simulink model "detector13"  (Simulink 2.20)
settings: Solver=FixedStepDiscrete  StartTime=0.0  StopTime=30  RelTol=1e-3  AbsTol=1e-6
undefined symbols (not defined in the file): firls, get
libraries: BufferedDSP x22, dspbuff x7, dspsnks x2, dsparch x2, WinAudio x1
settings Model: SaveTime=off  SaveOutput=off  ConsistencyChecking=off  RTWPlaceOutputsASAP=off  RTWTemplateMakefile=c:\nfc\matlab\simulink\grt_vc_sgm.tmf  RTWMakeCommand="make_rtw USER_SRCS=\"winmm.lib\" USER_INCLUDES=\"-Ic:\\nfc\\matlab\\Simulink\\BufferedDSP\\src\\rtw\""

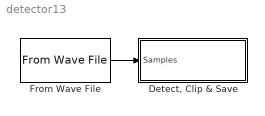
== system detector13 ==
  "Detect, Clip & Save" : Subsystem  mask(DetectClipNSave){buffersize=8192, f0=4100, f1=5500, threshold=2, numChannels=1, col_major=0, fs=22050}
      mask prompts: buffersize "Buffer Size:"; f0 "Lower Frequency (Hz):"; f1 "Upper Frequency (Hz):"; numChannels "Number of Channels:"; col_major "Column major channel order:"; fs "Sample Rate (Hz):"
      mask help: Detects acoustic events in a frequency band, clips, and saves them to disk.
      mask Help: Detects acoustic events in a frequency band, clips, and saves them to disk.
  From Wave File : WinAudio/From Wave File  sampleRate=22050  buffersize=8192  stereo=off  col_major=1  filename=c:\dicktest
  wires:
  From Wave File/1 -> "Detect, Clip & Save"/1(Samples)

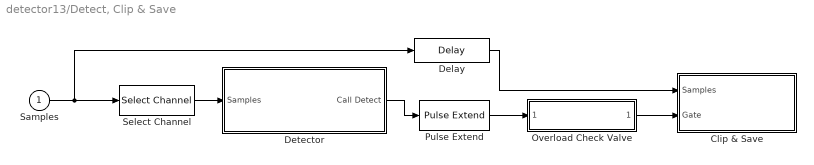
== system detector13/Detect, Clip & Save ==
  Samples : Inport  Port=1  PortWidth=buffersize * numChannels  SampleTime=-1
  Clip & Save : Subsystem  mask(ClipAndSave){buffersize=buffersize, fifosize=buffersize * 4, numChannels=numChannels, col_major=col_major, ftype=Wave, saveDir=c:\temp\calls, fname=Call, fnamestyle=Time from start, fs=fs}
      mask prompts: buffersize "Buffer size (samples):"; fifosize "FIFO size (samples):"; numChannels "Number of Channels:"; col_major "Column major channel order"; ftype "File type:"; saveDir "Save Directory:"; fname "File Name Prefix:"; fnamestyle "File name time stamp:"; fs "Sample Rate (Hz):"
      mask help: Clips sections from "Samples" according to "Gate" and saves to Save Directory using File Name Prefix and adding a time stamp.
      mask Help: Clips sections from "Samples" according to "Gate" and saves to Save Directory using File Name Prefix and adding a time stamp.
      mask StyleString: edit,edit,edit,edit,popup(Wave|Mac Binary|Matlab|ASCII Float|ASCII Fixed|Binary Float|Binary Fixed|AIFF),edit,edit,popup(GMT|Local time|Time from start),edit
  Delay : BufferedDSP/Memory/Delay  buffersize=buffersize  delay=15000  numChannels=numChannels  col_major=col_major
  Detector : Subsystem  mask(Detector){buffersize=buffersize, f0=f0, f1=f1, filterLength=100, threshold=threshold, numChannels=1, col_major=col_major, fs=fs}
      mask prompts: buffersize "Buffer Size:"; f0 "Lower Frequency (Hz):"; f1 "Upper Frequency (Hz):"; filterLength "Filter Length:"; numChannels "Number of Channels:"; col_major "Column major channel order:"; fs "Sample Rate:"
      mask help: Examines band-limited energy for events.
  Overload Check Valve : Subsystem  mask(Overload Check Valve){buffersize=buffersize, guardTime=20, numEvents=40, fs=fs}
      mask prompts: buffersize "Buffer size (samples):"; guardTime "Length of time to check: (sec)"; numEvents "Prohibited number of events:"; fs "Sample rate (Hz):"
      mask help: Input and output signals are single channel Boolean event markers. If more than a prohibited number of events occur in a specified time duration, the output is zero. Otherwise, the input is passed through (ANDed) to the output.
      mask Help: Input and output signals are single channel Boolean event markers.  If more than a prohibited number of events occur in a specified time duration, the output is zero.  Otherwise, the input is passed through (ANDed) to the output.
      mask Display: disp(sprintf('%d events in %d sec',numEvents,guardTime))
  Pulse Extend : BufferedDSP/Pulse Shapers/Pulse Extend  buffersize=buffersize  lag=10000  numChannels=1  col_major=col_major
  Select Channel : BufferedDSP/Multichannel/Select Channel  buffersize=buffersize  selectChannel=1  numChannels=numChannels  col_major=col_major
  wires:
  Detector/1(Call Detect) -> Pulse Extend/1
  Samples/1 -> Delay/1, Select Channel/1
  Select Channel/1 -> Detector/1(Samples)
  Delay/1 -> Clip & Save/1(Samples)
  Pulse Extend/1 -> Overload Check Valve/1("      ")
  Overload Check Valve/1("     ") -> Clip & Save/2(Gate)

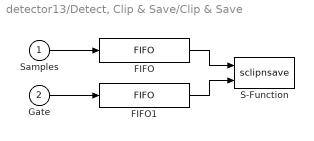
== system detector13/Detect, Clip & Save/Clip & Save ==
  Samples : Inport  Port=1  PortWidth=buffersize * numChannels  SampleTime=-1
  Gate : Inport  Port=2  PortWidth=buffersize  SampleTime=-1
  FIFO : BufferedDSP/Memory/FIFO  input_width=buffersize  output_width=fifosize  numChannels=numChannels  col_major=col_major
  FIFO1 : BufferedDSP/Memory/FIFO  input_width=buffersize  output_width=fifosize  numChannels=1  col_major=col_major
  S-Function : S-Function  FunctionName=sclipnsave  Parameters=buffersize fifosize numChannels col_major fname saveDir ftype fnamestyle fs  PortCounts=[]  SFunctionModules=''
  wires:
  FIFO1/1 -> S-Function/2
  FIFO/1 -> S-Function/1
  Gate/1 -> FIFO1/1
  Samples/1 -> FIFO/1

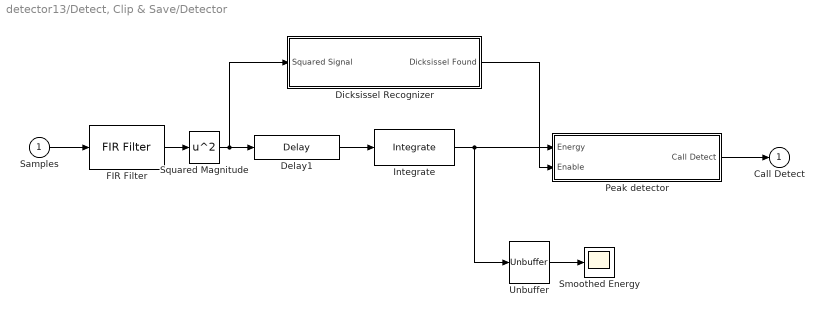
== system detector13/Detect, Clip & Save/Detector ==
  Samples : Inport  Port=1  PortWidth=buffersize *numChannels  SampleTime=-1
  Delay1 : BufferedDSP/Memory/Delay  buffersize=buffersize  delay=10000  numChannels=1  col_major=1
  Dicksissel Recognizer : Subsystem  mask{buffersize=8192, fs=22050, threshold=0.5, FilterLength=200}
      mask prompts: buffersize "Buffer size:"; fs "Sample Rate (Hz):"; FilterLength "Filter Length:"
  FIR Filter : BufferedDSP/Filter/Row Major/FIR Filter  input_width=buffersize  nfft_in=2*buffersize  h=firls(filterLength-1,[0 f0-100 f0 f1 f1+100 fs/2]/(fs/2),[0,0,1,1,0,0])  numChannels=numChannels
  Integrate : BufferedDSP/Filter/Integrate  buffersize=buffersize  integration_time=1103  normalize=on  initial_value=0  numChannels=numChannels  col_major=col_major
  Peak detector : Subsystem  mask(PeakDetector){threshold=threshold, buffersize=buffersize, numChannels=numChannels, col_major=col_major, fs=fs}
      mask prompts: buffersize "Buffer Size:"; numChannels "Number of Channels:"; col_major "Column major channel order:"; fs "Sample Rate:"
      mask help: Finds large plateaus in an energy signal.
      mask Help: Finds large plateaus in an energy signal.
  Smoothed Energy : Scope
      settings: TickLabels=on  TimeRange=auto  YMin=0  YMax=0.0004  SaveToWorkspace=off  SaveName=ScopeData  LimitMaxRows=off  Decimation=100
  Squared Magnitude : Math  Operator=square
  Unbuffer : dspbuff/Unbuffer  num_chans=1  Ts=buffersize/fs
  Call Detect : Outport  Port=1  InitialOutput=0
  wires:
  FIR Filter/1 -> Squared Magnitude/1
  Samples/1 -> FIR Filter/1
  Peak detector/1(Call Detect) -> Call Detect/1
  Squared Magnitude/1 -> Dicksissel Recognizer/1(Squared Signal), Delay1/1
  Dicksissel Recognizer/1(Dicksissel Found) -> Peak detector/2(Enable)
  Delay1/1 -> Integrate/1
  Unbuffer/1 -> Smoothed Energy/1
  Integrate/1 -> Peak detector/1(Energy), Unbuffer/1

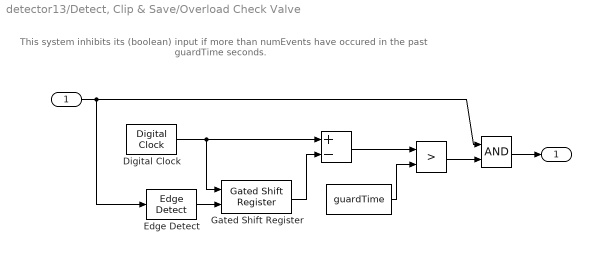
== system detector13/Detect, Clip & Save/Overload Check Valve ==
  note: This system inhibits its (boolean) input if
      | more than numEvents have occured
      | in the past guardTime seconds.
  "      " : Inport  Port=1  PortWidth=buffersize  SampleTime=-1
  " " : Constant  Value=guardTime
  "  " : RelationalOperator  Operator=>
  "    " : Logic  Operator=AND  Inputs=2
  "        " : Sum  Inputs=+-
  Digital Clock : BufferedDSP/Counters/Digital Clock  buffersize=buffersize  t0=guardTime+1  fs=fs
  Edge Detect : BufferedDSP/Pulse Shapers/Edge Detect  buffersize=buffersize  numChannels=1  col_major=1
  Gated Shift Register : BufferedDSP/Memory/Gated Shift Register  buffersize=buffersize  reg_size=numEvents  numChannels=1  col_major=1
  "     " : Outport  Port=1  InitialOutput=0
  wires:
  Digital Clock/1 -> Gated Shift Register/1, "        "/1
  Edge Detect/1 -> Gated Shift Register/2
  Gated Shift Register/1 -> "        "/2
  "        "/1 -> "  "/1
  " "/1 -> "  "/2
  "      "/1 -> "    "/1, Edge Detect/1
  "    "/1 -> "     "/1
  "  "/1 -> "    "/2

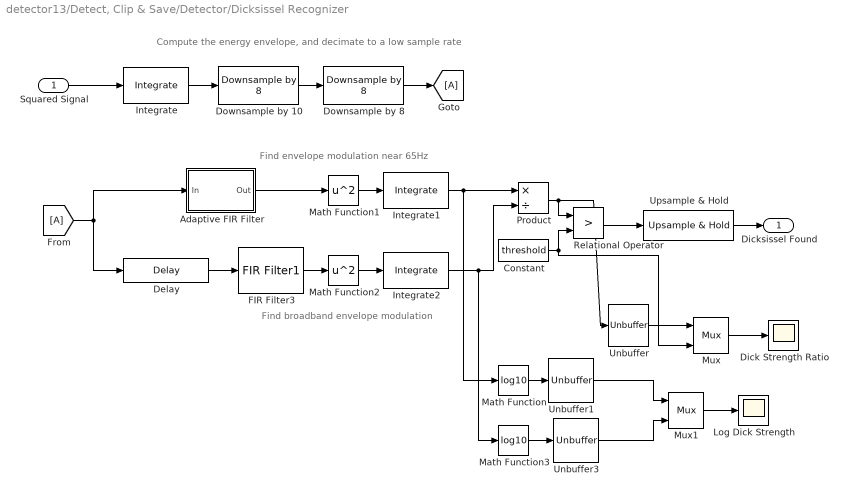
== system detector13/Detect, Clip & Save/Detector/Dicksissel Recognizer ==
  note: Find broadband envelope modulation
  note: Find envelope modulation near 65Hz
  note: Compute the energy envelope, and decimate to a low sample rate
  Squared Signal : Inport  Port=1  PortWidth=buffersize  SampleTime=-1
  Adaptive FIR Filter : Subsystem  mask(Adaptive Center Frequency Bandpass Filter){Bmin=55, Bmax=80, Bandwidth=18, mu=1e6, EnergyDuration=0.030, FilterLength=FilterLength, fs=fs/64, buffersize=buffersize/64}
      mask prompts: Bmin "Min Center Frequency: (Hz)"; Bmax "Max Center Frequency: (Hz)"; Bandwidth "Bandwidth: (Hz)"; mu "Adaption Gain:"; EnergyDuration "Energy Test Duration: (sec)"; FilterLength "Filter Length:"; fs "Sampling Frequency: (Hz)"; buffersize "Buffer Size:"
      mask help: A fixed-bandwidth adaptive center frequency bandpass FIR filter, that adapts the center frequency to maximize output power.
      mask init:
      | EnergyFilterLength=round(EnergyDuration*fs);
      | N=max([EnergyFilterLength,FilterLength]);
      mask Help: A fixed-bandwidth adaptive center frequency bandpass FIR filter, that adapts the center frequency to maximize output power.   The adaption gain determines how fast the center frequency changes.
  Constant : Constant  Value=threshold
  Delay : BufferedDSP/Memory/Delay  buffersize=buffersize/64  delay=2*buffersize/64  numChannels=1  col_major=1
  Dick Strength Ratio : Scope
      settings: TickLabels=on  TimeRange=auto  YMin=0  YMax=1  SaveToWorkspace=off  SaveName=ScopeData  LimitMaxRows=off
  Downsample by 10 : BufferedDSP/Filter/Single Channel/Downsample by 8  buffersize=buffersize  h=fir1(100,1/8)
  Downsample by 8 : BufferedDSP/Filter/Single Channel/Downsample by 8  buffersize=buffersize/8  h=fir1(100,1/8)
  FIR Filter3 : BufferedDSP/Filter/Row Major/FIR Filter1  input_width=buffersize/64  nfft_in=buffersize/32  h=fir1(FilterLength,[20,110]/(fs/128),'DC-0')  numChannels=1  Ts=buffersize/fs
  Integrate : BufferedDSP/Filter/Integrate  buffersize=buffersize  integration_time=100  normalize=on  initial_value=0  numChannels=1  col_major=0
  Integrate1 : BufferedDSP/Filter/Integrate  buffersize=buffersize/64  integration_time=round(0.600*fs/64)  normalize=on  initial_value=0  numChannels=1  col_major=0
  Integrate2 : BufferedDSP/Filter/Integrate  buffersize=buffersize/64  integration_time=round(0.600*fs/64)  normalize=on  initial_value=0  numChannels=1  col_major=0
  Log Dick Strength : Scope
      settings: TickLabels=on  TimeRange=auto  YMin=-15  YMax=-5  SaveToWorkspace=off  SaveName=ScopeData  LimitMaxRows=off
  Math Function : Math  Operator=log10
  Math Function1 : Math  Operator=square
  Math Function2 : Math  Operator=square
  Math Function3 : Math  Operator=log10
  Mux : Mux  Inputs=2
  Mux1 : Mux  Inputs=2
  Product : Product  Inputs=*/
  Relational Operator : RelationalOperator  Operator=>
  Unbuffer : dspbuff/Unbuffer  num_chans=1  Ts=buffersize/fs
  Unbuffer1 : dspbuff/Unbuffer  num_chans=1  Ts=buffersize/fs
  Unbuffer3 : dspbuff/Unbuffer  num_chans=1  Ts=buffersize/fs
  Upsample & Hold : BufferedDSP/Other/Upsample & Hold  buffersize=buffersize/64  L=64
  Dicksissel Found : Outport  Port=1
  wires:
  Downsample by 8/1 -> [A]
  Integrate/1 -> Downsample by 10/1
  Downsample by 10/1 -> Downsample by 8/1
  Squared Signal/1 -> Integrate/1
  [A] -> Adaptive FIR Filter/1(In), Delay/1
  FIR Filter3/1 -> Math Function2/1
  Mux/1 -> Dick Strength Ratio/1
  Unbuffer/1 -> Mux/1
  Math Function/1 -> Unbuffer1/1
  Mux1/1 -> Log Dick Strength/1
  Unbuffer1/1 -> Mux1/1
  Math Function3/1 -> Unbuffer3/1
  Unbuffer3/1 -> Mux1/2
  Math Function1/1 -> Integrate1/1
  Math Function2/1 -> Integrate2/1
  Integrate2/1 -> Product/2, Math Function3/1
  Integrate1/1 -> Product/1, Math Function/1
  Adaptive FIR Filter/1(Out) -> Math Function1/1
  Relational Operator/1 -> Upsample & Hold/1
  Upsample & Hold/1 -> Dicksissel Found/1
  Constant/1 -> Relational Operator/2, Mux/2
  Product/1 -> Relational Operator/1, Unbuffer/1
  Delay/1 -> FIR Filter3/1

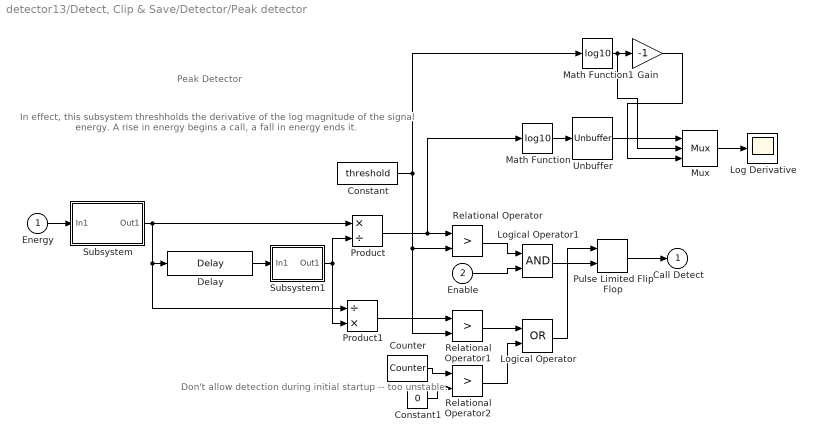
== system detector13/Detect, Clip & Save/Detector/Peak detector ==
  note: Don't allow detection during
      | initial startup -- too unstable.
  note: Peak Detector
  note: In effect, this subsystem threshholds
      | the derivative of the log magnitude
      | of the signal energy.  A rise in energy
      | begins a call, a fall in energy ends it.
  Energy : Inport  Port=1  PortWidth=buffersize * numChannels  SampleTime=-1
  Enable : Inport  Port=2  PortWidth=buffersize  SampleTime=-1
  Constant : Constant  Value=threshold
  Constant1 : Constant  Value=0
  Counter : BufferedDSP/Counters/Counter  buffersize=buffersize  initial_count=1.2*buffersize  count_direction=Down  has_stop_count=on  stop_count=0  numChannels=numChannels  col_major=1  ts=buffersize/fs
  Delay : BufferedDSP/Memory/Delay  buffersize=buffersize  delay=fix(fs * .020)  numChannels=numChannels  col_major=col_major
  Gain : Gain  Gain=-1
  Log Derivative : Scope
      settings: TickLabels=on  TimeRange=auto  YMin=-0.5  YMax=0.5  SaveToWorkspace=off  SaveName=ScopeData  LimitMaxRows=off  Decimation=100
  Logical Operator : Logic  Operator=OR  Inputs=2
  Logical Operator1 : Logic  Operator=AND  Inputs=2
  Math Function : Math  Operator=log10
  Math Function1 : Math  Operator=log10
  Mux : Mux  Inputs=3
  Product : Product  Inputs=*/
  Product1 : Product  Inputs=/*
  Pulse Limited Flip Flop : BufferedDSP/Memory/Pulse Limited Flip Flop  buffersize=buffersize  initial_state=0  minLimit=fix(0.1 * fs)  maxLimit=fix(0.4 * fs)  numChannels=numChannels  col_major=col_major
  Relational Operator : RelationalOperator  Operator=>
  Relational Operator1 : RelationalOperator  Operator=>
  Relational Operator2 : RelationalOperator  Operator=>
  Subsystem : Subsystem
      mask Type: Prevent divide-by-zero
      mask Display: disp('Prevent\n divide-by-zero')
  Subsystem1 : Subsystem
      mask Type: Prevent divide-by-zero
      mask Display: disp('Prevent\n divide-by-zero')
  Unbuffer : dspbuff/Unbuffer  num_chans=1  Ts=buffersize/fs
  Call Detect : Outport  Port=1  InitialOutput=0
  wires:
  Relational Operator2/1 -> Logical Operator/2
  Constant1/1 -> Relational Operator2/2
  Counter/1 -> Relational Operator2/1
  Relational Operator1/1 -> Logical Operator/1
  Product1/1 -> Relational Operator1/1
  Pulse Limited Flip Flop/1 -> Call Detect/1
  Logical Operator/1 -> Pulse Limited Flip Flop/1
  Relational Operator/1 -> Logical Operator1/1
  Enable/1 -> Logical Operator1/2
  Logical Operator1/1 -> Pulse Limited Flip Flop/2
  Subsystem1/1(Out1) -> Product/2, Product1/2
  Subsystem/1(Out1) -> Product/1, Delay/1, Product1/1
  Delay/1 -> Subsystem1/1(In1)
  Energy/1 -> Subsystem/1(In1)
  Math Function/1 -> Unbuffer/1
  Mux/1 -> Log Derivative/1
  Unbuffer/1 -> Mux/1
  Constant/1 -> Relational Operator/2, Relational Operator1/2, Math Function1/1
  Math Function1/1 -> Gain/1, Mux/2
  Gain/1 -> Mux/3
  Product/1 -> Relational Operator/1, Math Function/1

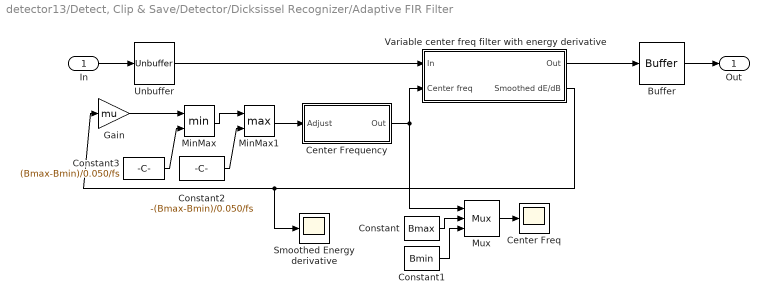
== system detector13/Detect, Clip & Save/Detector/Dicksissel Recognizer/Adaptive FIR Filter ==
  In : Inport  Port=1  PortWidth=-1  SampleTime=-1
  Buffer : dspbuff/Buffer  N=buffersize  V=0  Ts=1/fs  ic=0
  Center Freq : Scope
      settings: TickLabels=on  TimeRange=auto  YMin=55  YMax=80  SaveToWorkspace=off  SaveName=ScopeData  LimitMaxRows=off
  Center Frequency : Subsystem
  Constant : Constant  Value=Bmax
  Constant1 : Constant  Value=Bmin
  Constant2 : Constant  Value=-(Bmax-Bmin)/0.050/fs
  Constant3 : Constant  Value=(Bmax-Bmin)/0.050/fs
  Gain : Gain  Gain=mu
  MinMax : MinMax  Function=min  Inputs=2
  MinMax1 : MinMax  Function=max  Inputs=2
  Mux : Mux  Inputs=3
  Smoothed Energy derivative : Scope
      settings: TickLabels=on  TimeRange=auto  YMin=-0.001  YMax=0.001  SaveToWorkspace=off  SaveName=ScopeData  LimitMaxRows=off
  Unbuffer : dspbuff/Unbuffer  num_chans=1  Ts=buffersize/fs
  Variable center freq filter with energy derivative : Subsystem
  Out : Outport  Port=1
  wires:
  Variable center freq filter with energy derivative/1(Out) -> Buffer/1
  Mux/1 -> Center Freq/1
  Constant/1 -> Mux/2
  Constant1/1 -> Mux/3
  Center Frequency/1(Out) -> Variable center freq filter with energy derivative/2(Center freq), Mux/1
  Buffer/1 -> Out/1
  MinMax1/1 -> Center Frequency/1(Adjust)
  MinMax/1 -> MinMax1/1
  Constant2/1 -> MinMax1/2
  Constant3/1 -> MinMax/2
  In/1 -> Unbuffer/1
  Unbuffer/1 -> Variable center freq filter with energy derivative/1(In)
  Gain/1 -> MinMax/1
  Variable center freq filter with energy derivative/2(Smoothed dE/dB) -> Smoothed Energy derivative/1, Gain/1

== system detector13/Detect, Clip & Save/Detector/Peak detector/Subsystem ==
  In1 : Inport  Port=1  PortWidth=-1  SampleTime=-1
  Constant : Constant  Value=eps
  Sum : Sum  Inputs=++
  Out1 : Outport  Port=1
  wires:
  Sum/1 -> Out1/1
  Constant/1 -> Sum/2
  In1/1 -> Sum/1

== system detector13/Detect, Clip & Save/Detector/Peak detector/Subsystem1 ==
  In1 : Inport  Port=1  PortWidth=-1  SampleTime=-1
  Constant : Constant  Value=eps
  Sum : Sum  Inputs=++
  Out1 : Outport  Port=1
  wires:
  Sum/1 -> Out1/1
  Constant/1 -> Sum/2
  In1/1 -> Sum/1

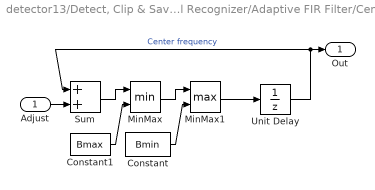
== system detector13/Detect, Clip & Save/Detector/Dicksissel Recognizer/Adaptive FIR Filter/Center Frequency ==
  Adjust : Inport  Port=1  PortWidth=-1  SampleTime=-1
  Constant : Constant  Value=Bmin
  Constant1 : Constant  Value=Bmax
  MinMax : MinMax  Function=min  Inputs=2
  MinMax1 : MinMax  Function=max  Inputs=2
  Sum : Sum  Inputs=++
  Unit Delay : UnitDelay  X0=(Bmax+Bmin)/2  SampleTime=-1
  Out : Outport  Port=1
  wires:
  MinMax1/1 -> Unit Delay/1
  MinMax/1 -> MinMax1/1
  Constant/1 -> MinMax1/2
  Constant1/1 -> MinMax/2
  Sum/1 -> MinMax/1
  Adjust/1 -> Sum/2
  Unit Delay/1 -> Out/1, Sum/1  "Center frequency"

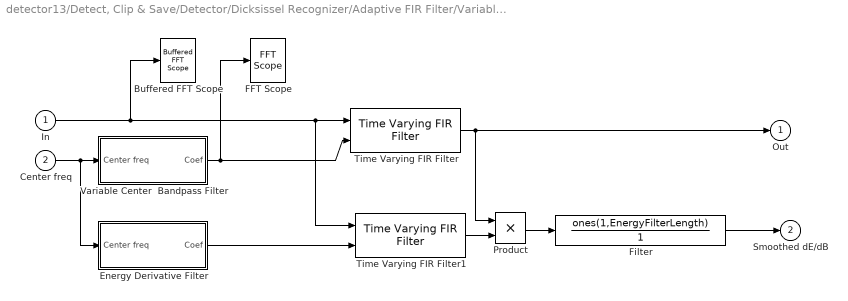
== system detector13/Detect, Clip & Save/Detector/Dicksissel Recognizer/Adaptive FIR Filter/Variable center freq filter with energy derivative ==
  In : Inport  Port=1  PortWidth=-1  SampleTime=-1
  Center freq : Inport  Port=2  PortWidth=-1  SampleTime=-1
  Buffered FFT Scope : dspsnks/Buffered FFT Scope  radsPop=Hertz  frange=Half  ampl_scale=Magnitude  bufsize=FilterLength  olap=FilterLength-1  fftlength=max([2^nextpow2(FilterLength),512])  ylabel=Magnitude  figpos=get(0,'DefaultFigurePosition')  ts=1/fs
  Energy Derivative Filter : Subsystem  mask(Variable Center Bandpass Filter){M=FilterLength, windowname=hamming, delta=Bandwidth, fs=fs}
      mask prompts: M "Filter length"; windowname "Window function"; delta "Bandwidth (Hz)"; fs "Sampling Frequency: (Hz)"
      mask init:
      | window=eval([windowname,'(M)']);
  FFT Scope : dspsnks/FFT Scope  radsPop=Hertz  frange=Half  ampl_scale=Magnitude  fftlength=256  ylabel=Magnitude  figpos=get(0,'DefaultFigurePosition')  ts=1/fs
  Filter : DiscreteFilter  Numerator=ones(1,EnergyFilterLength)  Denominator=1  SampleTime=1/fs
  Product : Product  Inputs=2
  Time Varying FIR Filter : dsparch/Time Varying FIR Filter  lenNUM=FilterLength  ic=0
  Time Varying FIR Filter1 : dsparch/Time Varying FIR Filter  lenNUM=FilterLength  ic=0
  Variable Center  Bandpass Filter : Subsystem  mask(Variable Center Bandpass Filter){M=FilterLength, windowname=hamming, delta=Bandwidth, fs=fs}
      mask prompts: M "Filter length"; windowname "Window function"; delta "Bandwidth (Hz)"; fs "Sampling Frequency: (Hz)"
      mask init:
      | window=eval([windowname,'(M)']);
  Out : Outport  Port=1  InitialOutput=0
  Smoothed dE/dB : Outport  Port=2  InitialOutput=0
  wires:
  Center freq/1 -> Energy Derivative Filter/1(Center freq), Variable Center  Bandpass Filter/1(Center freq)
  Variable Center  Bandpass Filter/1(Coef) -> FFT Scope/1, Time Varying FIR Filter/2
  In/1 -> Buffered FFT Scope/1, Time Varying FIR Filter/1, Time Varying FIR Filter1/1
  Energy Derivative Filter/1(Coef) -> Time Varying FIR Filter1/2
  Time Varying FIR Filter1/1 -> Product/2
  Filter/1 -> Smoothed dE/dB/1
  Product/1 -> Filter/1
  Time Varying FIR Filter/1 -> Out/1, Product/1

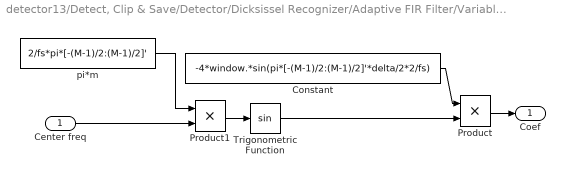
== system detector13/Detect, Clip & Save/Detector/Dicksissel Recognizer/Adaptive FIR Filter/Variable center freq filter with energy derivative/Energy Derivative Filter ==
  Center freq : Inport  Port=1  PortWidth=-1  SampleTime=-1
  Constant : Constant  Value=-4*window.*sin(pi*[-(M-1)/2:(M-1)/2]'*delta/2*2/fs)
  Product : Product  Inputs=2
  Product1 : Product  Inputs=2
  Trigonometric Function : Trigonometry  Operator=sin
  pi*m : Constant  Value=2/fs*pi*[-(M-1)/2:(M-1)/2]'
  Coef : Outport  Port=1  InitialOutput=0
  wires:
  Product1/1 -> Trigonometric Function/1
  pi*m/1 -> Product1/1
  Constant/1 -> Product/1
  Trigonometric Function/1 -> Product/2
  Center freq/1 -> Product1/2
  Product/1 -> Coef/1

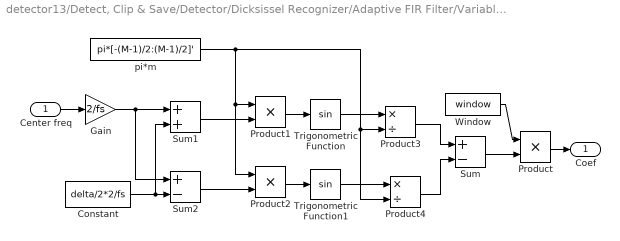
== system detector13/Detect, Clip & Save/Detector/Dicksissel Recognizer/Adaptive FIR Filter/Variable center freq filter with energy derivative/Variable Center  Bandpass Filter ==
  Center freq : Inport  Port=1  PortWidth=-1  SampleTime=-1
  Constant : Constant  Value=delta/2*2/fs
  Gain : Gain  Gain=2/fs
  Product : Product  Inputs=2
  Product1 : Product  Inputs=2
  Product2 : Product  Inputs=2
  Product3 : Product  Inputs=*/
  Product4 : Product  Inputs=*/
  Sum : Sum  Inputs=+-
  Sum1 : Sum  Inputs=++
  Sum2 : Sum  Inputs=+-
  Trigonometric Function : Trigonometry  Operator=sin
  Trigonometric Function1 : Trigonometry  Operator=sin
  Window : Constant  Value=window
  pi*m : Constant  Value=pi*[-(M-1)/2:(M-1)/2]'
  Coef : Outport  Port=1  InitialOutput=0
  wires:
  Constant/1 -> Sum1/2, Sum2/2
  Trigonometric Function/1 -> Product3/1
  Trigonometric Function1/1 -> Product4/1
  Product1/1 -> Trigonometric Function/1
  Product2/1 -> Trigonometric Function1/1
  pi*m/1 -> Product3/2, Product4/2, Product1/1, Product2/1
  Sum1/1 -> Product1/2
  Sum2/1 -> Product2/2
  Product/1 -> Coef/1
  Window/1 -> Product/1
  Sum/1 -> Product/2
  Product3/1 -> Sum/1
  Product4/1 -> Sum/2
  Gain/1 -> Sum1/1, Sum2/1
  Center freq/1 -> Gain/1
